simulink model "Lab2_prac_sim"  (R2019b)
settings: Solver=VariableStepAuto  StartTime=0.0  StopTime=Tfin  MaxStep=Tstep  RelTol=1e-3
values from neighbouring files (symbols this model uses):
  C = [1, 0, 0]    [Lab2_prac.m]
  x0 = [0, 0, 0]    [Lab2_prac.m]
undefined symbols (not defined in the file or in its folder): chua_fg, u_chua
libraries: cstblocks x1
settings Model: Creator=user  LastModifiedBy=user

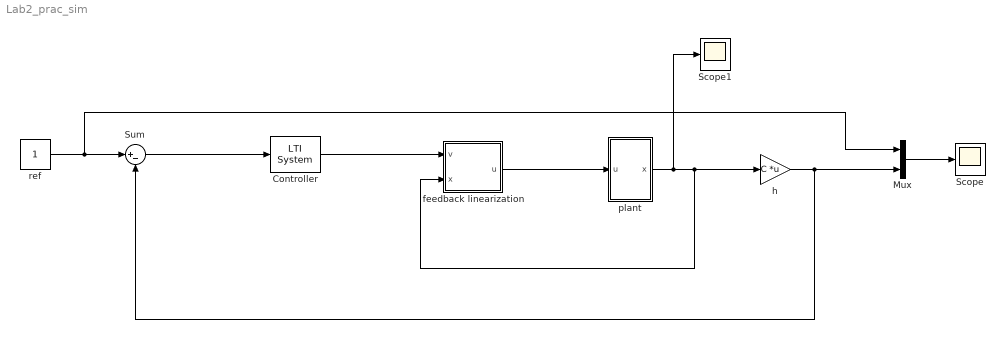
== system Lab2_prac_sim ==
  Controller : cstblocks/LTI System  sys=K  IC=[]
  Mux : Mux  Inputs=2
  Scope : Scope
  Scope1 : Scope
  Sum : Sum  Inputs=|+-
  feedback linearization : Subsystem
  h : Gain  Gain=C  Multiplication=Matrix(K*u)
  plant : Subsystem
  ref : Constant
  wires:
  feedback linearization/1(u) -> plant/1(u)
  plant/1(x) -> Scope1/1, feedback linearization/2(x), h/1
  h/1 -> Mux/2, Sum/2
  Mux/1 -> Scope/1
  Controller/1 -> feedback linearization/1(v)
  ref/1 -> Mux/1, Sum/1
  Sum/1 -> Controller/1

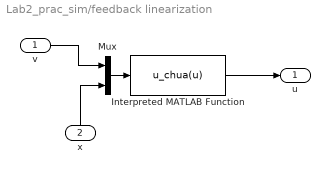
== system Lab2_prac_sim/feedback linearization ==
  v : Inport
  x : Inport  Port=2
  Interpreted MATLAB Function : MATLABFcn  MATLABFcn=u_chua(u)
  Mux : Mux  Inputs=2
  u : Outport  VectorParamsAs1DForOutWhenUnconnected=off
  wires:
  x/1 -> Mux/2
  Mux/1 -> Interpreted MATLAB Function/1
  v/1 -> Mux/1
  Interpreted MATLAB Function/1 -> u/1

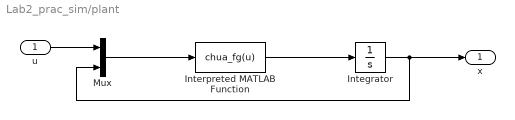
== system Lab2_prac_sim/plant ==
  u : Inport
  Integrator : Integrator  InitialCondition=x0
  Interpreted MATLAB Function : MATLABFcn  MATLABFcn=chua_fg(u)
  Mux : Mux  Inputs=2
  x : Outport
  wires:
  Mux/1 -> Interpreted MATLAB Function/1
  Integrator/1 -> x/1, Mux/2
  u/1 -> Mux/1
  Interpreted MATLAB Function/1 -> Integrator/1
